simulink model "kalman"  (R2015b)
settings: Solver=FixedStepDiscrete  StartTime=0.0  StopTime=10.0  FixedStep=T  RelTol=1e-3
InitFcn:
  | param
values from neighbouring files (symbols this model uses):
  T = 0.1    [param.m]
undefined symbols (not defined in the file or in its folder): DiscIntNeverNeededParam
libraries: commchan3 x1, simulink x1
settings Model: Creator=mishuk  LastModifiedBy=mishuk
settings DataIOCC: SaveFormat=Array
settings OptimizationCC: ExpressionDepthLimit=2147483647
settings DebuggingCC: UnderspecifiedInitializationDetection=Classic  MergeDetectMultiDrivingBlocksExec=none  SolverPrmCheckMsg=warning  StateNameClashWarn=warning
settings HardwareCC: ProdBitPerPointer=32  ProdLargestAtomicFloat=None  ProdIntDivRoundTo=Undefined  ProdEndianess=Unspecified  ProdWordSize=32  ProdHWDeviceType=32-bit Generic
settings RTWCC: GenCodeOnly=on
settings GRTTargetCC: GeneratePreprocessorConditionals=Disable all
settings ConfigComp: CovModelRefEnable=Off

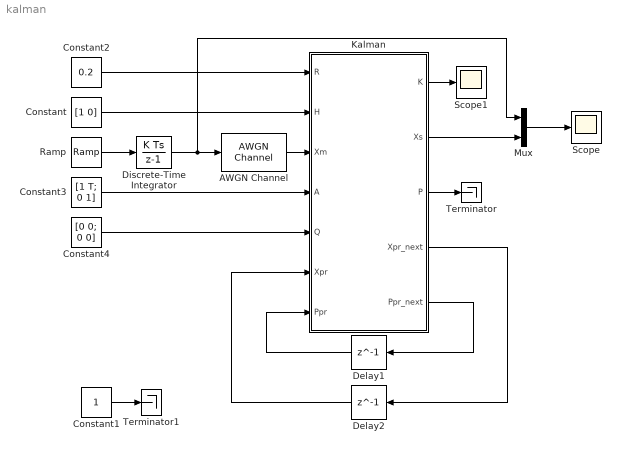
== system kalman ==
  AWGN Channel : commchan3/AWGN Channel  InputProcessing=Columns as channels (frame based)  seed=67  noiseMode=Variance from mask  EbNodB=10  EsNodB=10  SNRdB=10  bitsPerSym=1  Ps=1  Tsym=1  variance=noiseVariance
  Constant : Constant  Value=[1 0]  VectorParams1D=off  SampleTime=-1
  Constant1 : Constant  SampleTime=-1
  Constant2 : Constant  Value=0.2  SampleTime=-1
  Constant3 : Constant  Value=[1 T; 0 1]  SampleTime=-1
  Constant4 : Constant  Value=[0 0; 0 0]  SampleTime=-1
  Delay1 : Delay  DelayLength=1  InitialCondition=eye(2)
  Delay2 : Delay  DelayLength=1  InitialCondition=[0; 0]
  Discrete-Time Integrator : DiscreteIntegrator  gainval=1  InitialConditionSetting=State (most efficient)  SampleTime=T  ICPrevOutput=DiscIntNeverNeededParam  ICPrevScaledInput=DiscIntNeverNeededParam
  Kalman : MATLAB Function  TreatAsAtomicUnit=on
  Mux : Mux  Inputs=2
  Ramp : simulink/Sources/Ramp  slope=1  start=0  X0=0  VectorParams1D=off
  Scope : Scope
  Scope1 : Scope
  Terminator : Terminator
  Terminator1 : Terminator
  wires:
  Kalman/5(Ppr_next) -> Delay1/1
  Delay1/1 -> Kalman/7(Ppr)
  Kalman/4(Xpr_next) -> Delay2/1
  Delay2/1 -> Kalman/6(Xpr)
  Kalman/3(P) -> Terminator/1
  Kalman/1(K) -> Scope1/1
  Constant/1 -> Kalman/2(H)
  Constant2/1 -> Kalman/1(R)
  Constant3/1 -> Kalman/4(A)
  AWGN Channel/1 -> Kalman/3(Xm)
  Constant1/1 -> Terminator1/1
  Ramp/1 -> Discrete-Time Integrator/1
  Discrete-Time Integrator/1 -> Mux/1, AWGN Channel/1
  Kalman/2(Xs) -> Mux/2
  Mux/1 -> Scope/1
  Constant4/1 -> Kalman/5(Q)

== matlab function kalman/Kalman ==
  data: R input; H input; Xm input; A input; Q input; Xpr input; K output; Ppr input; Xs output; P output; Xpr_next output; Ppr_next output
function [K, Xs, P, Xpr_next, Ppr_next] = kalman(R, H, Xm, A, Q, Xpr, Ppr)

%% estimation
K = Ppr*H'*(R+H*Ppr*H')^(-1);
Xs = Xpr + K*(Xm-H*Xpr);
I = eye(length(Xpr));
P = (I - K*H)*Ppr + Q;

%% prediction
Xpr_next = A*Xs;
Ppr_next = A*P*A';
